simulink model "MagLev_Nonlinear"  (R2015b)
settings: Solver=VariableStepAuto  StartTime=0.0  StopTime=10.0  RelTol=1e-3
InitFcn:
  | a1 = 46.5894;
  | a2 = 0.007;
  | Kf = 5.0678e-6;
  | Ka = 11.7858;
  | Kl = 0.0065;
  | m = 1.1;
  | R = 1.1;
  | Ic = 1;
  | g = 9.81;
settings Model: Creator=Peter  LastModifiedBy=Peter

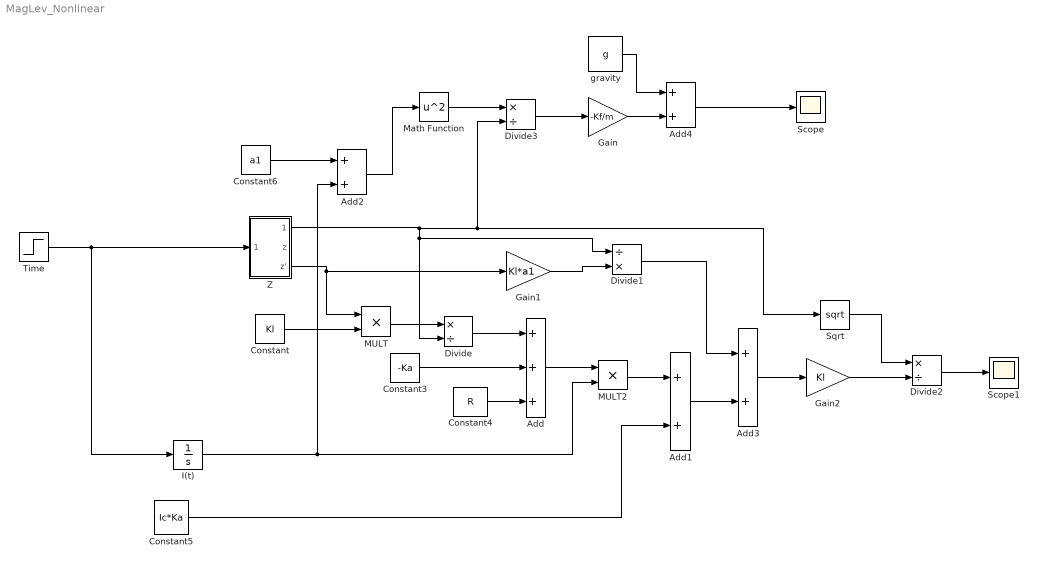
== system MagLev_Nonlinear ==
  Add : Sum  Inputs=+++
  Add{1..4} (4 alike) : Sum
  Constant : Constant  Value=Kl
  Constant3 : Constant  Value=-Ka
  Constant4 : Constant  Value=R
  Constant5 : Constant  Value=Ic*Ka
  Constant6 : Constant  Value=a1
  Divide : Product  Inputs=*/
  Divide1 : Product  Inputs=/*
  Divide2 : Product  Inputs=*/
  Divide3 : Product  Inputs=*/
  Gain : Gain  Gain=-Kf/m
  Gain1 : Gain  Gain=Kl*a1
  Gain2 : Gain  Gain=Kl
  I(t) : Integrator
  MULT : Product  Inputs=**
  MULT2 : Product  Inputs=**
  Math Function : Math  Operator=square  SaturateOnIntegerOverflow=on
  Scope : Scope
  Scope1 : Scope
  Sqrt : Sqrt  SaturateOnIntegerOverflow=on
  Time : Step  Time=5  SampleTime=0
  Z : Subsystem
  gravity : Constant  Value=g
  wires:
  Time/1 -> I(t)/1, Z/1(In1)
  Z/3(z') -> Gain1/1, MULT/1
  I(t)/1 -> Add2/2, MULT2/2
  Constant/1 -> MULT/2
  MULT/1 -> Divide/1
  Z/1((a2+z)^2) -> Divide3/2, Sqrt/1, Divide1/1, Divide/2
  Divide/1 -> Add/1
  Constant3/1 -> Add/2
  Constant4/1 -> Add/3
  Add/1 -> MULT2/1
  MULT2/1 -> Add1/1
  Constant5/1 -> Add1/2
  Gain1/1 -> Divide1/2
  Add1/1 -> Add3/2
  Divide1/1 -> Add3/1
  Add3/1 -> Gain2/1
  Gain2/1 -> Divide2/2
  Sqrt/1 -> Divide2/1
  Divide2/1 -> Scope1/1
  Constant6/1 -> Add2/1
  Add2/1 -> Math Function/1
  Math Function/1 -> Divide3/1
  Divide3/1 -> Gain/1
  Gain/1 -> Add4/2
  gravity/1 -> Add4/1
  Add4/1 -> Scope/1

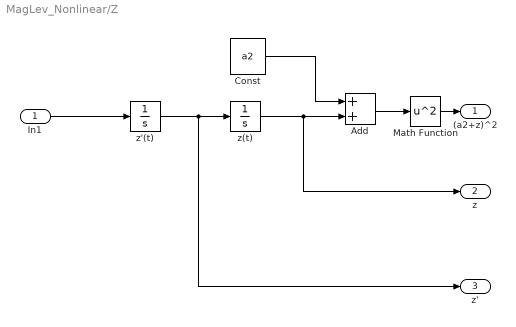
== system MagLev_Nonlinear/Z ==
  In1 : Inport
  Add : Sum
  Const : Constant  Value=a2
  Math Function : Math  Operator=square  SaturateOnIntegerOverflow=on
  z'(t) : Integrator
  z(t) : Integrator
  (a2+z)^2 : Outport
  z : Outport  Port=2
  z' : Outport  Port=3
  wires:
  z'(t)/1 -> z'/1, z(t)/1
  Const/1 -> Add/1
  In1/1 -> z'(t)/1
  Add/1 -> Math Function/1
  z(t)/1 -> z/1, Add/2
  Math Function/1 -> (a2+z)^2/1
